simulink model "dfilt1"  (R2021b)
settings: Solver=VariableStepAuto  StartTime=0.0  StopTime=4  MaxStep=1e-5  RelTol=1e-3
libraries: simulink x1
settings Model: Creator=Len_comp  LastModifiedBy=alexey
settings SolverCC: AlgebraicLoopSolver=TrustRegion
settings DebuggingCC: SFMachineParentedDataDiag=warning

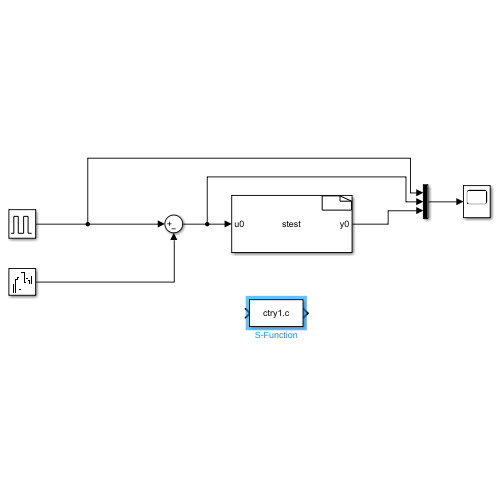
[thumbnail: Simulink's stored preview of the top-level diagram]
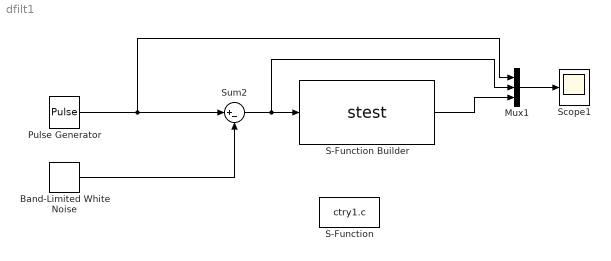
== system dfilt1 ==
  Band-Limited White Noise : simulink/Sources/Band-Limited White Noise  Cov=[0.005]  Ts=0.001  seed=[23341506453219]
  Mux1 : Mux  Inputs=3
  Pulse Generator : DiscretePulseGenerator  PulseType=Time based  Amplitude=6.5  Period=0.125  PulseWidth=50
  S-Function : S-Function  FunctionName=ctry1.c  SFunctionDeploymentMode=off  EnableBusSupport=off
  S-Function Builder : S-Function  FunctionName=stest  SFunctionModules=stest_wrapper  SFunctionDeploymentMode=off  EnableBusSupport=off  mask(S-Function Builder){}
      mask help: Simulink:masks:SFunctionBuilder_MD
      mask init:
      | val = [[.9  0.75 0.75 1 1 .9 .9 1]',[1 1 0.75 0.75 .9 .9 1 .9]'];try , sys = get_param(gcb,'SfunBuilderFcnName');if isempty(sys), sys = get_param(gcb,'FunctionName'); end,catch, sys = get_param(gcb,'FunctionName'); end
      settings: CopyFcn=set_param(gcbh,'LinkStatus','none')  OpenFcn=sfunctionwizard(gcbh)
      mask Display: plot(val(:,1),val(:,2)),disp(sys),port_label('input',1,'u0'),port_label('output',1,'y0')
  Scope1 : Scope
  Sum2 : Sum  Inputs=|+-
  wires:
  Pulse Generator/1 -> Mux1/1, Sum2/1
  Mux1/1 -> Scope1/1
  S-Function Builder/1 -> Mux1/3
  Sum2/1 -> S-Function Builder/1, Mux1/2
  Band-Limited White Noise/1 -> Sum2/2
